simulink model "motorControlWBT_zumo"  (R2014b)
settings: Solver=FixedStepDiscrete  SolverMode=SingleTasking  StartTime=0.0  StopTime=10.0  FixedStep=0.1  RelTol=1e-3
libraries: ZumoBotLib x1, arduinolib x1
settings Model: ExtModeTrigDuration=2  Creator=agajjar  LastModifiedBy=sandip
settings OptimizationCC: OptimizeModelRefInitCode=on  LifeSpan=1
settings DebuggingCC: UnderspecifiedInitializationDetection=Classic  MergeDetectMultiDrivingBlocksExec=none  SolverPrmCheckMsg=none
settings HardwareCC: ProdBitPerInt=16  ProdBitPerPointer=8  ProdIntDivRoundTo=Zero  ProdEndianess=LittleEndian  ProdWordSize=8  ProdHWDeviceType=Atmel->AVR
settings RTWCC: SystemTargetFile=realtime.tlc  GenerateMakefile=off  TemplateMakefile=realtime.tmf  Description=Run on Target Hardware  RTWVerbose=off  ProcessScript=realtime_make_rtw_hook
settings STFCustomTargetCC: TargetLibSuffix=.a  GenerateSampleERTMain=on  ERTCustomFileBanners=on  SupportNonInlinedSFcns=off  SupportVariableSizeSignals=on  MATLABClassNameForMDSCustomization=Simulink.SoftwareTarget.ERTCustomization  GRTInterface=off  SystemTargetFile=realtime.tlc
settings ERTTargetCC: GenerateSampleERTMain=on  ParMdlRefBuildCompliant=off  CompOptLevelCompliant=off  ConcurrentExecutionCompliant=off  CombineOutputUpdateFcns=off  ERTFirstTimeCompliant=off  SupportContinuousTime=on  SupportVariableSizeSignals=on  ModelStepFunctionPrototypeControlCompliant=off  CPPClassGenCompliant=off  ExtModeTransport=3  ExtModeMexFile=ext_serial_win32_comm  ExtModeMexArgs=0 1 9600  InlinedParameterPlacement=NonHierarchical  ERTSrcFileBannerTemplate=realtime_code_template.cgt  ERTHdrFileBannerTemplate=realtime_code_template.cgt  ERTDataSrcFileTemplate=realtime_code_template.cgt  ERTDataHdrFileTemplate=realtime_code_template.cgt  ERTCustomFileTemplate=realtime_file_process.tlc

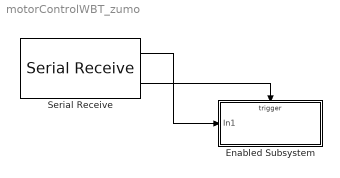
== system motorControlWBT_zumo ==
  Enabled Subsystem : Subsystem  TreatAsAtomicUnit=on
  Serial Receive : arduinolib/Serial Receive  portNumber=0  showOutStatus=on  sampleTime=0.1  blockPlatform=arduino
  wires:
  Serial Receive/1 -> Enabled Subsystem/1(In1)
  Serial Receive/2 -> Enabled Subsystem/Trigger

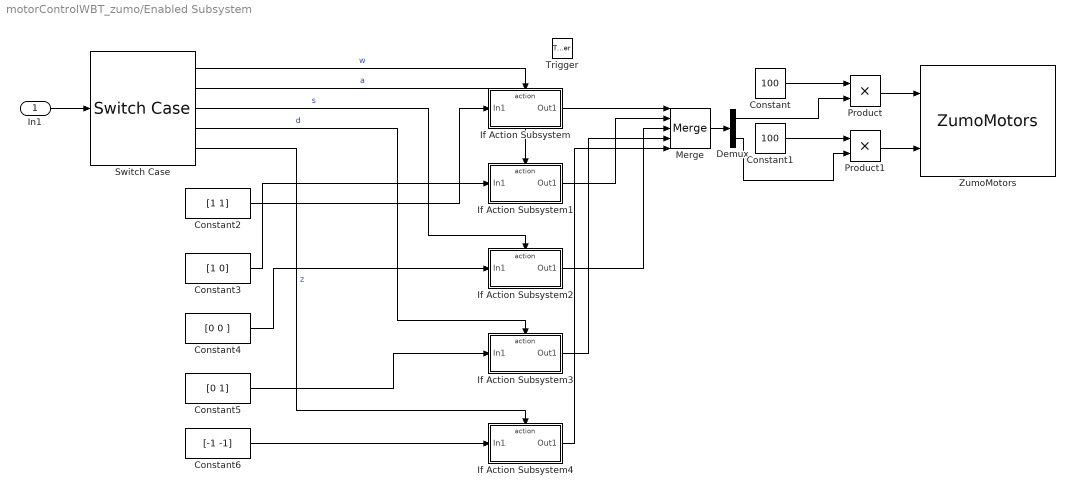
== system motorControlWBT_zumo/Enabled Subsystem ==
  In1 : Inport
  Trigger : TriggerPort  PortDimensions=1
  Constant : Constant  Value=100
  Constant1 : Constant  Value=100
  Constant2 : Constant  Value=[1 1]
  Constant3 : Constant  Value=[1 0]
  Constant4 : Constant  Value=[0 0 ]
  Constant5 : Constant  Value=[0 1]
  Constant6 : Constant  Value=[-1 -1]
  Demux : Demux  Outputs=2
  If Action Subsystem : Subsystem  TreatAsAtomicUnit=on
  If Action Subsystem1 : Subsystem  TreatAsAtomicUnit=on
  If Action Subsystem2 : Subsystem  TreatAsAtomicUnit=on
  If Action Subsystem3 : Subsystem  TreatAsAtomicUnit=on
  If Action Subsystem4 : Subsystem  TreatAsAtomicUnit=on
  Merge : Merge  Inputs=5
  Product : Product
  Product1 : Product
  Switch Case : SwitchCase  CaseConditions={119, 97, 115, 100, 122}  ShowDefaultCase=off
  ZumoMotors : ZumoBotLib/ZumoMotors  flipLeft=off  flipRight=off
  wires:
  In1/1 -> Switch Case/1
  Product/1 -> ZumoMotors/1
  Constant/1 -> Product/1
  Constant1/1 -> Product1/1
  Product1/1 -> ZumoMotors/2
  Merge/1 -> Demux/1
  Demux/1 -> Product/2
  Demux/2 -> Product1/2
  If Action Subsystem/1(Out1) -> Merge/1
  If Action Subsystem1/1(Out1) -> Merge/2
  If Action Subsystem2/1(Out1) -> Merge/3
  If Action Subsystem3/1(Out1) -> Merge/4
  If Action Subsystem4/1(Out1) -> Merge/5
  Switch Case/1 -> If Action Subsystem/Action  "w"
  Switch Case/2 -> If Action Subsystem1/Action  "a"
  Switch Case/3 -> If Action Subsystem2/Action  "s"
  Switch Case/4 -> If Action Subsystem3/Action  "d"
  Switch Case/5 -> If Action Subsystem4/Action  "z"
  Constant6/1 -> If Action Subsystem4/1(In1)
  Constant5/1 -> If Action Subsystem3/1(In1)
  Constant4/1 -> If Action Subsystem2/1(In1)
  Constant3/1 -> If Action Subsystem1/1(In1)
  Constant2/1 -> If Action Subsystem/1(In1)

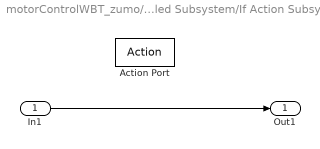
== system motorControlWBT_zumo/Enabled Subsystem/If Action Subsystem ==
  In1 : Inport
  Action Port : ActionPort  ActionType=case
  Out1 : Outport
  wires:
  In1/1 -> Out1/1

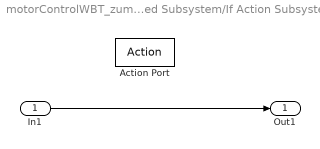
== system motorControlWBT_zumo/Enabled Subsystem/If Action Subsystem1 ==
  In1 : Inport
  Action Port : ActionPort  ActionType=case
  Out1 : Outport
  wires:
  In1/1 -> Out1/1

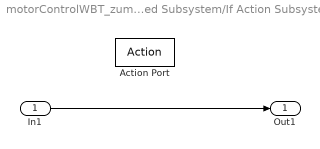
== system motorControlWBT_zumo/Enabled Subsystem/If Action Subsystem2 ==
  In1 : Inport
  Action Port : ActionPort  ActionType=case
  Out1 : Outport
  wires:
  In1/1 -> Out1/1

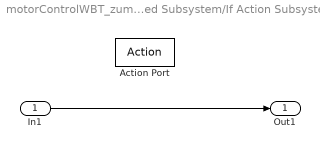
== system motorControlWBT_zumo/Enabled Subsystem/If Action Subsystem3 ==
  In1 : Inport
  Action Port : ActionPort  ActionType=case
  Out1 : Outport
  wires:
  In1/1 -> Out1/1

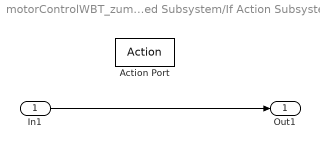
== system motorControlWBT_zumo/Enabled Subsystem/If Action Subsystem4 ==
  In1 : Inport
  Action Port : ActionPort  ActionType=case
  Out1 : Outport
  wires:
  In1/1 -> Out1/1
